simulink model "GotoviiShema"  (R2025b)
settings: Solver=VariableStepAuto  StartTime=0.0  StopTime=10.0  RelTol=1e-3
undefined symbols (not defined in the file): ki, kp
settings Model: Creator=Krist  LastModifiedBy=Krist

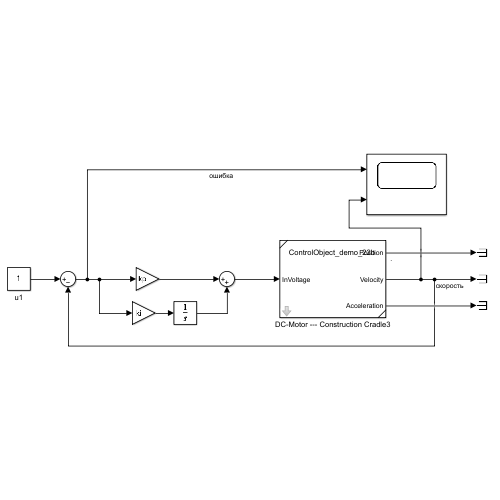
[thumbnail: Simulink's stored preview of the top-level diagram]
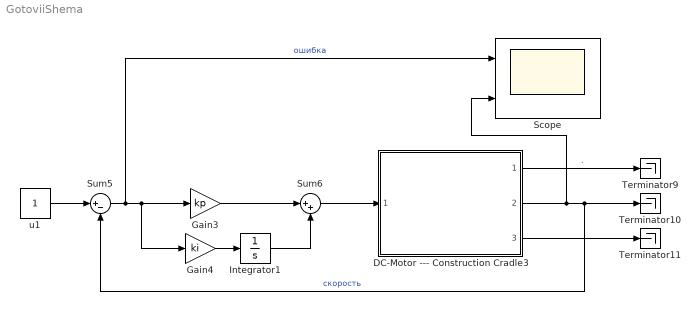
== system GotoviiShema ==
  DC-Motor --- Construction Cradle3 : Subsystem  ReferencedSubsystem=ControlObject_demo_22b  L=2.06*10^(-3)  R=11.6  km=85.8*10^(-3)  kw=111  J_motor=19.7*10^(-4)  vis_friction_coef_motor=0.001  i_gear=80  J_gear=0.001  vis_friction_coef_gear=0.001  r_wheel=0.1  J_wheel=5  vis_friction_coef_cradle=0.001  veh_mass=20  alpha=5
  Gain3 : Gain  Gain=kp
  Gain4 : Gain  Gain=ki
  Integrator1 : Integrator
  Scope : Scope  NumInputPorts=2
      settings: ActiveDisplayYMinimum=-0.30405347582002507  ActiveDisplayYMaximum=1.3216019167459
  Sum5 : Sum  Inputs=|+-
  Sum6 : Sum  Inputs=|++
  Terminator10 : Terminator
  Terminator11 : Terminator
  Terminator9 : Terminator
  u1 : Constant
  wires:
  Gain3/1 -> Sum6/1
  Sum6/1 -> DC-Motor --- Construction Cradle3/1
  DC-Motor --- Construction Cradle3/3 -> Terminator11/1
  u1/1 -> Sum5/1
  DC-Motor --- Construction Cradle3/2 -> Scope/2, Sum5/2, Terminator10/1  "скорость"
  Sum5/1 -> Scope/1, Gain3/1, Gain4/1  "ошибка"
  DC-Motor --- Construction Cradle3/1 -> Terminator9/1  "."
  Integrator1/1 -> Sum6/2
  Gain4/1 -> Integrator1/1
